simulink model "un2_2"  (R2020a)
settings: Solver=ode113  StartTime=0.0  StopTime=time  FixedStep=0.05  RelTol=1e-10
values from neighbouring files (symbols this model uses):
  g = 9.81    [lab2.m]
  Kd = 100    [lab2.m]
  Kp = 10    [lab2.m]
  th1 = 3.1    [lab2.m]
  th2 = 9.5    [lab2.m]
  th3 = 0.24    [lab2.m]
  th4 = 0.77    [lab2.m]
settings Model: Creator=ajankowi  LastModifiedBy=adamj

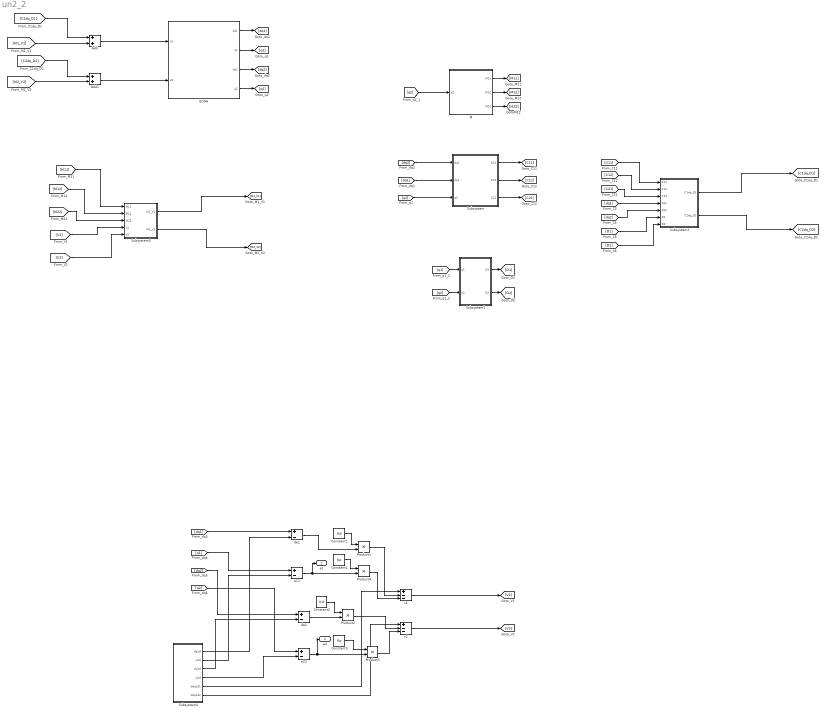
== system un2_2 ==
  Add : Sum
  Add1 : Sum
  Constant1 : Constant  Value=Kd
  Constant2 : Constant  Value=Kd
  Constant3 : Constant  Value=Kp
  Constant4 : Constant  Value=Kp
  EDDA : Subsystem
  M : Subsystem
  Product{1..4} (4 alike) : Product
  Subsystem : Subsystem
  Subsystem1 : Subsystem
  Subsystem2 : Subsystem
  Subsystem3 : Subsystem
  Subsystem4 : Subsystem
  de1 : Sum  Inputs=+-
  de2 : Sum  Inputs=+-
  e11 : Sum  Inputs=+-
  e22 : Sum  Inputs=+-
  v1 : Sum  Inputs=+--
  v2 : Sum  Inputs=+--
  e1 : Outport
  e2 : Outport  Port=2
  wires:
  Add/1 -> EDDA/1(U1`)
  Add1/1 -> EDDA/2(U2)
  M/3(M22) -> [M22]
  M/1(M11) -> [M11]
  [q2] -> M/1(q2)
  M/2(M12) -> [M12]
  EDDA/4(q2) -> [q2]
  Subsystem1/2(D2) -> [D2]
  [q1] -> Subsystem1/1(q1)
  Subsystem/1(C11) -> [C11]
  Subsystem/3(C21) -> [C21]
  [dq2] -> Subsystem/1(dq2)
  Subsystem1/1(D1) -> [D1]
  [q2] -> Subsystem1/2(q2)
  [q2] -> Subsystem/3(q2)
  Subsystem/2(C12) -> [C12]
  [dq1] -> Subsystem/2(dq1)
  EDDA/1(dq1) -> [dq1]
  EDDA/2(q1) -> [q1]
  EDDA/3(dq2) -> [dq2]
  Subsystem2/1(C1dq_D1) -> [C1dq_D1]
  Subsystem2/2(C2dq_D2) -> [C2dq_D2]
  [C11] -> Subsystem2/1(C11)
  [C12] -> Subsystem2/2(C12)
  [C21] -> Subsystem2/3(C21)
  [dq1] -> Subsystem2/4(dq1)
  [dq2] -> Subsystem2/5(dq2)
  [D1] -> Subsystem2/6(D1)
  [D2] -> Subsystem2/7(D2)
  [C1dq_D1] -> Add/1
  [C2dq_D2] -> Add1/1
  [M2_V2] -> Add1/2
  [M1_V1] -> Add/2
  Subsystem3/1(M1_V1) -> [M1_V1]
  Subsystem3/2(M2_V2) -> [M2_V2]
  [M11] -> Subsystem3/1(M11)
  [M12] -> Subsystem3/2(M12)
  [M22] -> Subsystem3/3(M22)
  [V1] -> Subsystem3/4(V1)
  [V2] -> Subsystem3/5(V2)
  Subsystem4/5(ddq1d1) -> v1/1
  Subsystem4/6(ddq1d2) -> v2/1
  Constant1/1 -> Product1/1
  Product1/1 -> v1/2
  [dq1] -> de1/1
  Subsystem4/1(dq1d) -> de1/2
  de1/1 -> Product1/2
  v1/1 -> [V1]
  [q1] -> e11/1
  Subsystem4/2(q1d) -> e11/2
  Constant4/1 -> Product4/1
  e11/1 -> e1/1, Product4/2
  Product4/1 -> v1/3
  v2/1 -> [V2]
  [dq2] -> de2/1
  Subsystem4/3(dq2d) -> de2/2
  [q2] -> e22/1
  Subsystem4/4(q2d) -> e22/2
  Constant2/1 -> Product2/1
  de2/1 -> Product2/2
  Product2/1 -> v2/2
  Constant3/1 -> Product3/1
  e22/1 -> e2/1, Product3/2
  Product3/1 -> v2/3

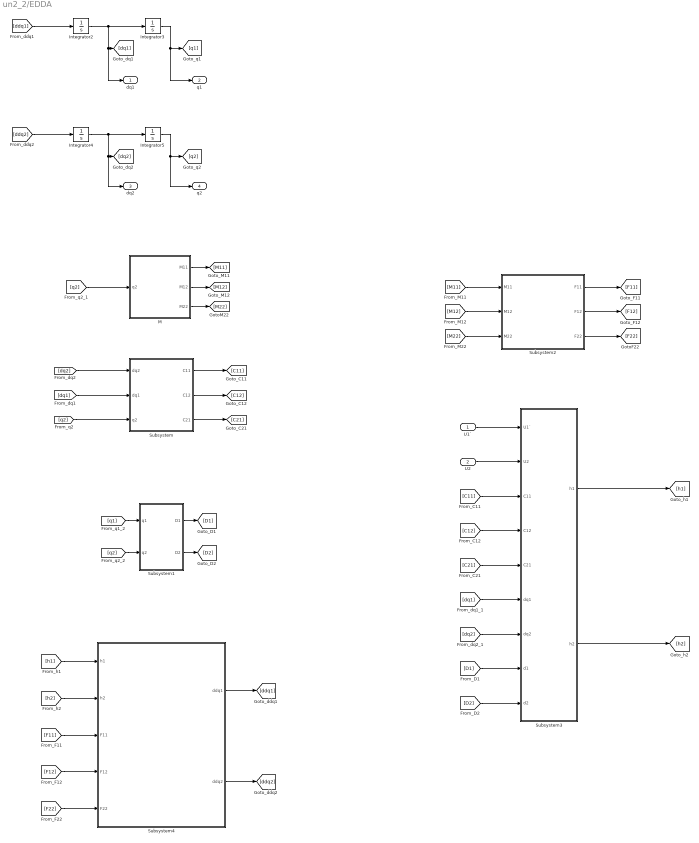
== system un2_2/EDDA ==
  U1` : Inport
  U2 : Inport  Port=2
  Integrator{2..5} (4 alike) : Integrator
  M : Subsystem
  Subsystem : Subsystem
  Subsystem1 : Subsystem
  Subsystem2 : Subsystem
  Subsystem3 : Subsystem
  Subsystem4 : Subsystem
  dq1 : Outport
  q1 : Outport  Port=2
  dq2 : Outport  Port=3
  q2 : Outport  Port=4
  wires:
  [dq1] -> Subsystem/2(dq1)
  [q2] -> M/1(q2)
  [ddq2] -> Integrator4/1
  [D1] -> Subsystem3/8(d1)
  Integrator4/1 -> dq2/1, [dq2], Integrator5/1
  Subsystem/3(C21) -> [C21]
  [q2] -> Subsystem1/2(q2)
  Integrator2/1 -> dq1/1, [dq1], Integrator3/1
  [M22] -> Subsystem2/3(M22)
  Subsystem3/2(h2) -> [h2]
  Subsystem4/2(ddq2) -> [ddq2]
  [D2] -> Subsystem3/9(d2)
  Subsystem4/1(ddq1) -> [ddq1]
  [F11] -> Subsystem4/3(F11)
  [q1] -> Subsystem1/1(q1)
  Subsystem2/1(F11) -> [F11]
  Subsystem2/2(F12) -> [F12]
  [dq2] -> Subsystem3/7(dq2)
  [C12] -> Subsystem3/4(C12)
  [q2] -> Subsystem/3(q2)
  Subsystem1/1(D1) -> [D1]
  [h2] -> Subsystem4/2(h2)
  U1`/1 -> Subsystem3/1(U1`)
  M/1(M11) -> [M11]
  Integrator5/1 -> q2/1, [q2]
  [C21] -> Subsystem3/5(C21)
  Integrator3/1 -> q1/1, [q1]
  [dq1] -> Subsystem3/6(dq1)
  [M12] -> Subsystem2/2(M12)
  [ddq1] -> Integrator2/1
  [M11] -> Subsystem2/1(M11)
  [dq2] -> Subsystem/1(dq2)
  M/2(M12) -> [M12]
  U2/1 -> Subsystem3/2(U2)
  Subsystem/2(C12) -> [C12]
  [C11] -> Subsystem3/3(C11)
  M/3(M22) -> [M22]
  Subsystem/1(C11) -> [C11]
  Subsystem1/2(D2) -> [D2]
  Subsystem2/3(F22) -> [F22]
  [F22] -> Subsystem4/5(F22)
  [h1] -> Subsystem4/1(h1)
  [F12] -> Subsystem4/4(F12)
  Subsystem3/1(h1) -> [h1]

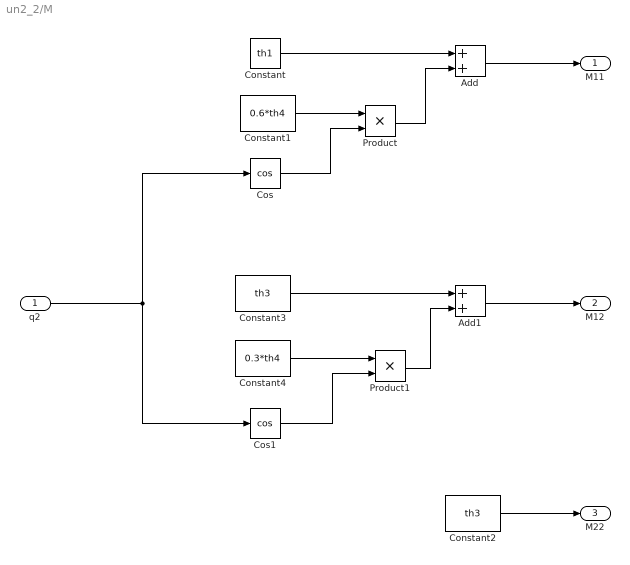
== system un2_2/M ==
  q2 : Inport
  Add : Sum
  Add1 : Sum
  Constant : Constant  Value=th1
  Constant1 : Constant  Value=0.6*th4
  Constant2 : Constant  Value=th3
  Constant3 : Constant  Value=th3
  Constant4 : Constant  Value=0.3*th4
  Cos : Trigonometry  Operator=cos
  Cos1 : Trigonometry  Operator=cos
  Product : Product
  Product1 : Product
  M11 : Outport
  M12 : Outport  Port=2
  M22 : Outport  Port=3
  wires:
  q2/1 -> Cos/1, Cos1/1
  Constant/1 -> Add/1
  Product/1 -> Add/2
  Constant1/1 -> Product/1
  Add/1 -> M11/1
  Cos/1 -> Product/2
  Constant2/1 -> M22/1
  Add1/1 -> M12/1
  Constant3/1 -> Add1/1
  Constant4/1 -> Product1/1
  Cos1/1 -> Product1/2
  Product1/1 -> Add1/2

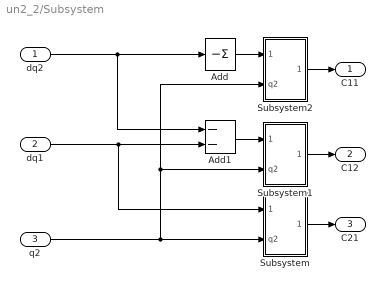
== system un2_2/Subsystem ==
  dq2 : Inport
  dq1 : Inport  Port=2
  q2 : Inport  Port=3
  Add : Sum  Inputs=-
  Add1 : Sum  Inputs=--
  Subsystem : Subsystem
  Subsystem1 : Subsystem
  Subsystem2 : Subsystem
  C11 : Outport
  C12 : Outport  Port=2
  C21 : Outport  Port=3
  wires:
  dq2/1 -> Add1/1, Add/1
  dq1/1 -> Subsystem/1(in1), Add1/2
  q2/1 -> Subsystem2/2(q2), Subsystem1/2(q2), Subsystem/2(q2)
  Subsystem/1(out2) -> C21/1
  Add1/1 -> Subsystem1/1(in1)
  Subsystem1/1(out2) -> C12/1
  Subsystem2/1(out2) -> C11/1
  Add/1 -> Subsystem2/1(in1)

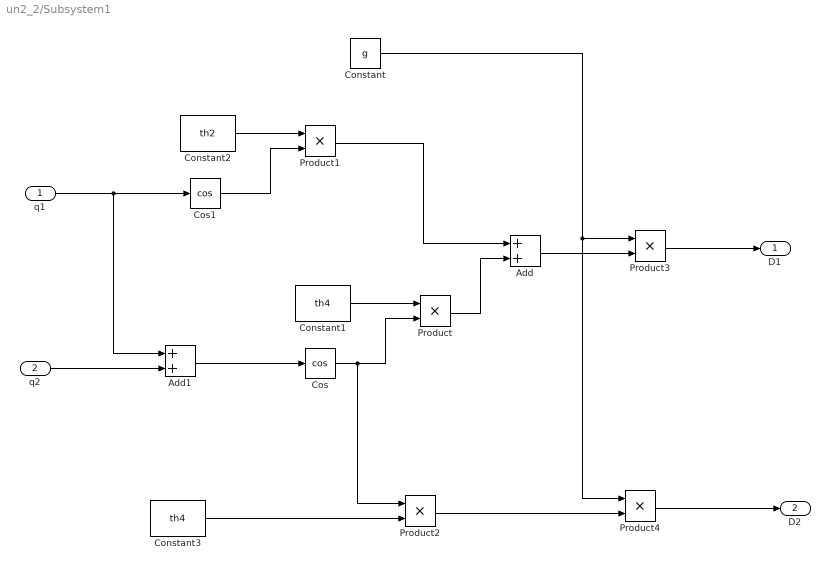
== system un2_2/Subsystem1 ==
  q1 : Inport
  q2 : Inport  Port=2
  Add : Sum
  Add1 : Sum
  Constant : Constant  Value=g
  Constant1 : Constant  Value=th4
  Constant2 : Constant  Value=th2
  Constant3 : Constant  Value=th4
  Cos : Trigonometry  Operator=cos
  Cos1 : Trigonometry  Operator=cos
  Product{,1..4} (5 alike) : Product
  D1 : Outport
  D2 : Outport  Port=2
  wires:
  q2/1 -> Add1/2
  Constant2/1 -> Product1/1
  Constant1/1 -> Product/1
  Cos/1 -> Product2/1, Product/2
  q1/1 -> Add1/1, Cos1/1
  Product1/1 -> Add/1
  Product/1 -> Add/2
  Cos1/1 -> Product1/2
  Constant3/1 -> Product2/2
  Add1/1 -> Cos/1
  Product3/1 -> D1/1
  Add/1 -> Product3/2
  Constant/1 -> Product4/1, Product3/1
  Product2/1 -> Product4/2
  Product4/1 -> D2/1

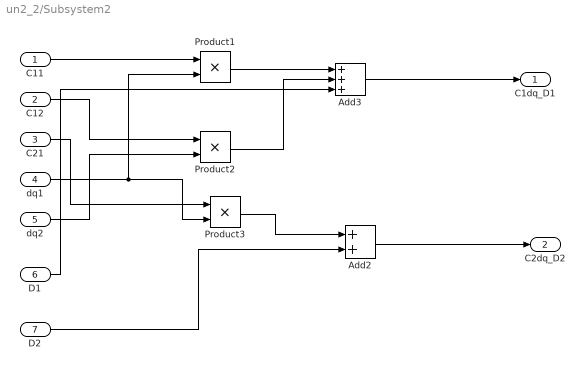
== system un2_2/Subsystem2 ==
  C11 : Inport
  C12 : Inport  Port=2
  C21 : Inport  Port=3
  dq1 : Inport  Port=4
  dq2 : Inport  Port=5
  D1 : Inport  Port=6
  D2 : Inport  Port=7
  Add2 : Sum
  Add3 : Sum  Inputs=+++
  Product1 : Product
  Product2 : Product
  Product3 : Product
  C1dq_D1 : Outport
  C2dq_D2 : Outport  Port=2
  wires:
  C11/1 -> Product1/1
  D1/1 -> Add3/3
  dq1/1 -> Product3/2, Product1/2
  C21/1 -> Product3/1
  D2/1 -> Add2/2
  Product1/1 -> Add3/1
  Add3/1 -> C1dq_D1/1
  Product2/1 -> Add3/2
  dq2/1 -> Product2/2
  C12/1 -> Product2/1
  Product3/1 -> Add2/1
  Add2/1 -> C2dq_D2/1

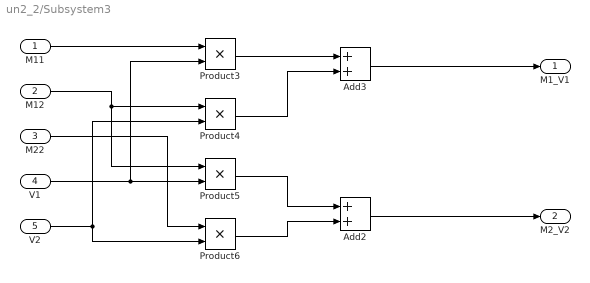
== system un2_2/Subsystem3 ==
  M11 : Inport
  M12 : Inport  Port=2
  M22 : Inport  Port=3
  V1 : Inport  Port=4
  V2 : Inport  Port=5
  Add2 : Sum
  Add3 : Sum
  Product{3..6} (4 alike) : Product
  M1_V1 : Outport
  M2_V2 : Outport  Port=2
  wires:
  M22/1 -> Product6/1
  M12/1 -> Product5/1, Product4/1
  Product5/1 -> Add2/1
  V2/1 -> Product6/2, Product4/2
  Add2/1 -> M2_V2/1
  V1/1 -> Product5/2, Product3/2
  M11/1 -> Product3/1
  Add3/1 -> M1_V1/1
  Product3/1 -> Add3/1
  Product6/1 -> Add2/2
  Product4/1 -> Add3/2

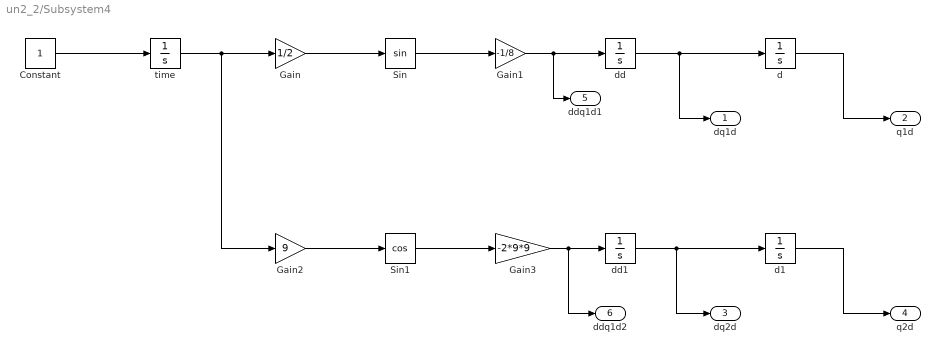
== system un2_2/Subsystem4 ==
  Constant : Constant
  Gain : Gain  Gain=1/2
  Gain1 : Gain  Gain=-1/8
  Gain2 : Gain  Gain=9
  Gain3 : Gain  Gain=-2*9*9
  Sin : Trigonometry
  Sin1 : Trigonometry  Operator=cos
  d : Integrator
  d1 : Integrator  InitialCondition=2
  dd : Integrator  InitialCondition=1/4
  dd1 : Integrator
  time : Integrator
  dq1d : Outport
  q1d : Outport  Port=2
  dq2d : Outport  Port=3
  q2d : Outport  Port=4
  ddq1d1 : Outport  Port=5
  ddq1d2 : Outport  Port=6
  wires:
  dd/1 -> dq1d/1, d/1
  Constant/1 -> time/1
  dd1/1 -> dq2d/1, d1/1
  Sin/1 -> Gain1/1
  Sin1/1 -> Gain3/1
  time/1 -> Gain2/1, Gain/1
  d/1 -> q1d/1
  Gain2/1 -> Sin1/1
  d1/1 -> q2d/1
  Gain1/1 -> ddq1d1/1, dd/1
  Gain3/1 -> ddq1d2/1, dd1/1
  Gain/1 -> Sin/1

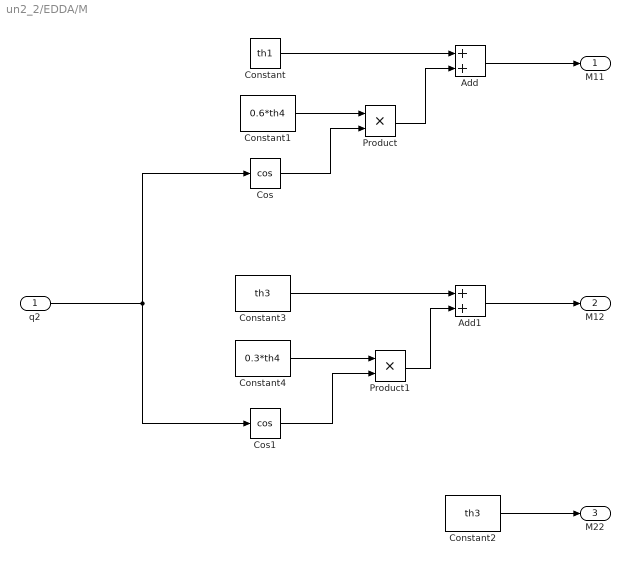
== system un2_2/EDDA/M ==
  q2 : Inport
  Add : Sum
  Add1 : Sum
  Constant : Constant  Value=th1
  Constant1 : Constant  Value=0.6*th4
  Constant2 : Constant  Value=th3
  Constant3 : Constant  Value=th3
  Constant4 : Constant  Value=0.3*th4
  Cos : Trigonometry  Operator=cos
  Cos1 : Trigonometry  Operator=cos
  Product : Product
  Product1 : Product
  M11 : Outport
  M12 : Outport  Port=2
  M22 : Outport  Port=3
  wires:
  q2/1 -> Cos/1, Cos1/1
  Constant/1 -> Add/1
  Product/1 -> Add/2
  Constant1/1 -> Product/1
  Add/1 -> M11/1
  Cos/1 -> Product/2
  Constant2/1 -> M22/1
  Add1/1 -> M12/1
  Constant3/1 -> Add1/1
  Constant4/1 -> Product1/1
  Cos1/1 -> Product1/2
  Product1/1 -> Add1/2

== system un2_2/EDDA/Subsystem ==
  dq2 : Inport
  dq1 : Inport  Port=2
  q2 : Inport  Port=3
  Add : Sum  Inputs=-
  Add1 : Sum  Inputs=--
  Subsystem : Subsystem
  Subsystem1 : Subsystem
  Subsystem2 : Subsystem
  C11 : Outport
  C12 : Outport  Port=2
  C21 : Outport  Port=3
  wires:
  dq2/1 -> Add1/1, Add/1
  dq1/1 -> Subsystem/1(in1), Add1/2
  q2/1 -> Subsystem2/2(q2), Subsystem1/2(q2), Subsystem/2(q2)
  Subsystem/1(out2) -> C21/1
  Add1/1 -> Subsystem1/1(in1)
  Subsystem1/1(out2) -> C12/1
  Subsystem2/1(out2) -> C11/1
  Add/1 -> Subsystem2/1(in1)

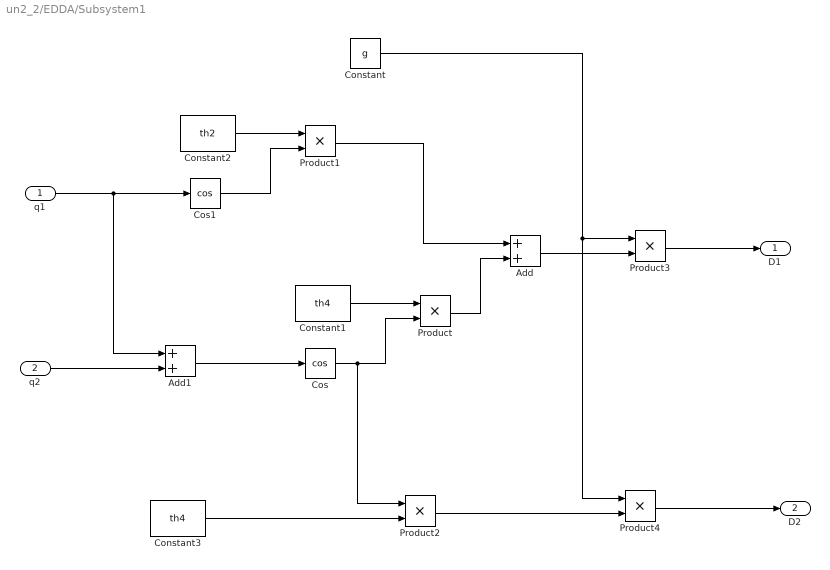
== system un2_2/EDDA/Subsystem1 ==
  q1 : Inport
  q2 : Inport  Port=2
  Add : Sum
  Add1 : Sum
  Constant : Constant  Value=g
  Constant1 : Constant  Value=th4
  Constant2 : Constant  Value=th2
  Constant3 : Constant  Value=th4
  Cos : Trigonometry  Operator=cos
  Cos1 : Trigonometry  Operator=cos
  Product{,1..4} (5 alike) : Product
  D1 : Outport
  D2 : Outport  Port=2
  wires:
  q2/1 -> Add1/2
  Constant2/1 -> Product1/1
  Constant1/1 -> Product/1
  Cos/1 -> Product2/1, Product/2
  q1/1 -> Add1/1, Cos1/1
  Product1/1 -> Add/1
  Product/1 -> Add/2
  Cos1/1 -> Product1/2
  Constant3/1 -> Product2/2
  Add1/1 -> Cos/1
  Product3/1 -> D1/1
  Add/1 -> Product3/2
  Constant/1 -> Product4/1, Product3/1
  Product2/1 -> Product4/2
  Product4/1 -> D2/1

== system un2_2/EDDA/Subsystem2 ==
  M11 : Inport
  M12 : Inport  Port=2
  M22 : Inport  Port=3
  Add : Sum  Inputs=-
  Divide : Product  Inputs=*/
  Divide1 : Product  Inputs=*/
  Divide2 : Product  Inputs=*/
  detM : MATLAB Function  TreatAsAtomicUnit=on
  F11 : Outport
  F12 : Outport  Port=2
  F22 : Outport  Port=3
  wires:
  M11/1 -> Divide1/1, detM/1(M11)
  Divide1/1 -> F22/1
  Add/1 -> F12/1
  detM/1(detM) -> Divide1/2, Divide2/2, Divide/2
  M22/1 -> Divide/1, detM/3(M22)
  M12/1 -> Divide2/1, detM/2(M12)
  Divide/1 -> F11/1
  Divide2/1 -> Add/1

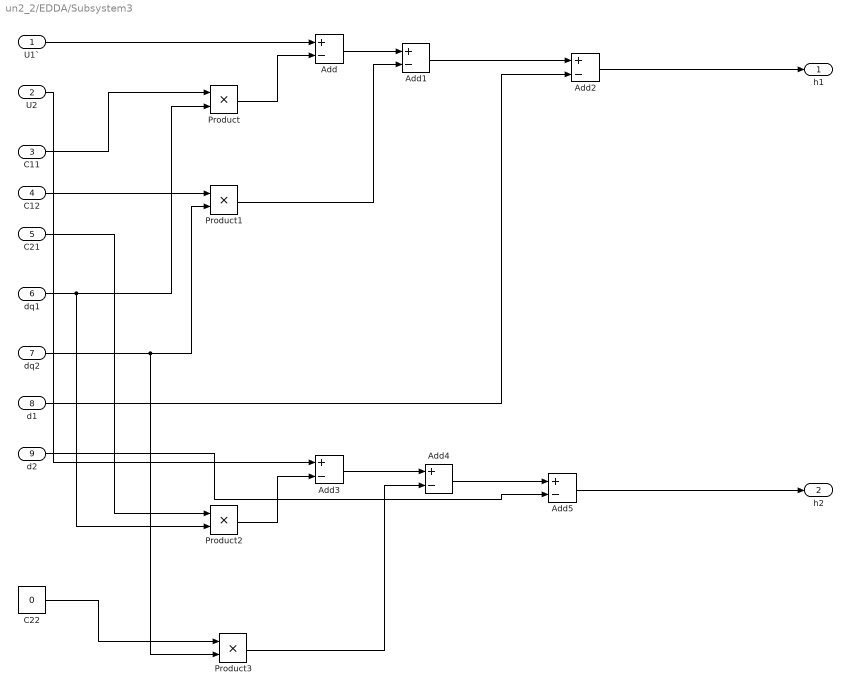
== system un2_2/EDDA/Subsystem3 ==
  U1` : Inport
  U2 : Inport  Port=2
  C11 : Inport  Port=3
  C12 : Inport  Port=4
  C21 : Inport  Port=5
  dq1 : Inport  Port=6
  dq2 : Inport  Port=7
  d1 : Inport  Port=8
  d2 : Inport  Port=9
  Add{,1..5} (6 alike) : Sum  Inputs=+-
  C22 : Constant  Value=0
  Product{,1..3} (4 alike) : Product
  h1 : Outport
  h2 : Outport  Port=2
  wires:
  Product/1 -> Add/2
  Add5/1 -> h2/1
  dq1/1 -> Product2/2, Product/2
  Add2/1 -> h1/1
  Add/1 -> Add1/1
  U1`/1 -> Add/1
  dq2/1 -> Product3/2, Product1/2
  C12/1 -> Product1/1
  d1/1 -> Add2/2
  Product3/1 -> Add4/2
  Product2/1 -> Add3/2
  Add1/1 -> Add2/1
  Product1/1 -> Add1/2
  d2/1 -> Add5/2
  C11/1 -> Product/1
  Add4/1 -> Add5/1
  U2/1 -> Add3/1
  Add3/1 -> Add4/1
  C21/1 -> Product2/1
  C22/1 -> Product3/1

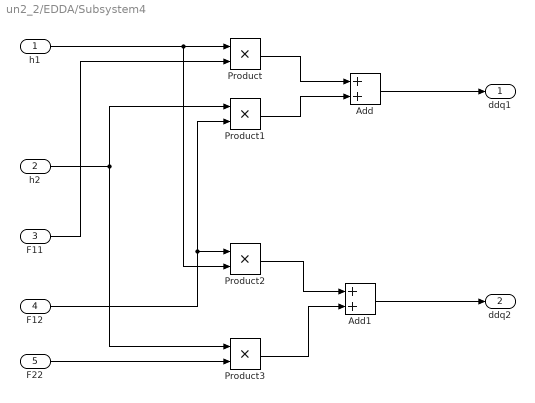
== system un2_2/EDDA/Subsystem4 ==
  h1 : Inport
  h2 : Inport  Port=2
  F11 : Inport  Port=3
  F12 : Inport  Port=4
  F22 : Inport  Port=5
  Add : Sum
  Add1 : Sum
  Product{,1..3} (4 alike) : Product
  ddq1 : Outport
  ddq2 : Outport  Port=2
  wires:
  h2/1 -> Product1/1, Product3/1
  Product1/1 -> Add/2
  F12/1 -> Product2/1, Product1/2
  Add1/1 -> ddq2/1
  Add/1 -> ddq1/1
  h1/1 -> Product2/2, Product/1
  F11/1 -> Product/2
  Product2/1 -> Add1/1
  F22/1 -> Product3/2
  Product3/1 -> Add1/2
  Product/1 -> Add/1

== system un2_2/Subsystem/Subsystem ==
  in1 : Inport
  q2 : Inport  Port=2
  Constant : Constant  Value=0.3*th4
  Product : Product
  Product1 : Product
  Trigonometric Function : Trigonometry
  out2 : Outport
  wires:
  Product1/1 -> out2/1
  in1/1 -> Product/2
  Trigonometric Function/1 -> Product1/1
  q2/1 -> Trigonometric Function/1
  Product/1 -> Product1/2
  Constant/1 -> Product/1

== system un2_2/Subsystem/Subsystem1 ==
  in1 : Inport
  q2 : Inport  Port=2
  Constant : Constant  Value=0.3*th4
  Product : Product
  Product1 : Product
  Trigonometric Function : Trigonometry
  out2 : Outport
  wires:
  Product1/1 -> out2/1
  in1/1 -> Product/2
  Trigonometric Function/1 -> Product1/1
  q2/1 -> Trigonometric Function/1
  Product/1 -> Product1/2
  Constant/1 -> Product/1

== system un2_2/Subsystem/Subsystem2 ==
  in1 : Inport
  q2 : Inport  Port=2
  Constant : Constant  Value=0.3*th4
  Product : Product
  Product1 : Product
  Trigonometric Function : Trigonometry
  out2 : Outport
  wires:
  Product1/1 -> out2/1
  in1/1 -> Product/2
  Trigonometric Function/1 -> Product1/1
  q2/1 -> Trigonometric Function/1
  Product/1 -> Product1/2
  Constant/1 -> Product/1

== system un2_2/EDDA/Subsystem/Subsystem ==
  in1 : Inport
  q2 : Inport  Port=2
  Constant : Constant  Value=0.3*th4
  Product : Product
  Product1 : Product
  Trigonometric Function : Trigonometry
  out2 : Outport
  wires:
  Product1/1 -> out2/1
  in1/1 -> Product/2
  Trigonometric Function/1 -> Product1/1
  q2/1 -> Trigonometric Function/1
  Product/1 -> Product1/2
  Constant/1 -> Product/1

== system un2_2/EDDA/Subsystem/Subsystem1 ==
  in1 : Inport
  q2 : Inport  Port=2
  Constant : Constant  Value=0.3*th4
  Product : Product
  Product1 : Product
  Trigonometric Function : Trigonometry
  out2 : Outport
  wires:
  Product1/1 -> out2/1
  in1/1 -> Product/2
  Trigonometric Function/1 -> Product1/1
  q2/1 -> Trigonometric Function/1
  Product/1 -> Product1/2
  Constant/1 -> Product/1

== system un2_2/EDDA/Subsystem/Subsystem2 ==
  in1 : Inport
  q2 : Inport  Port=2
  Constant : Constant  Value=0.3*th4
  Product : Product
  Product1 : Product
  Trigonometric Function : Trigonometry
  out2 : Outport
  wires:
  Product1/1 -> out2/1
  in1/1 -> Product/2
  Trigonometric Function/1 -> Product1/1
  q2/1 -> Trigonometric Function/1
  Product/1 -> Product1/2
  Constant/1 -> Product/1

== matlab function un2_2/EDDA/Subsystem2/detM ==
  data: M11 input; detM output; M12 input; M22 input
function detM = fcn(M11, M12, M22)

detM = (M11*M22)-(M12^2);
